simulink model "qdr_ct_test"  (R2012b)
settings: Solver=ode45  StartTime=0.0  StopTime=50000  RelTol=1e-3
libraries: xbsIndex_r4 x1070, casper_library_misc x5, xps_library x4, casper_library_delays x4
(part 2 of 10)

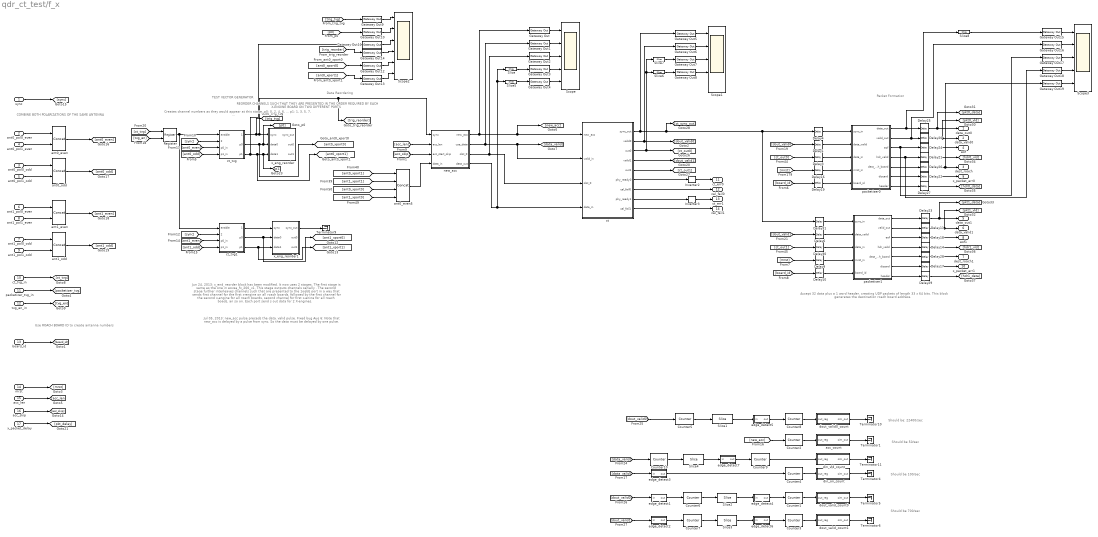
== system qdr_ct_test/f_x ==
  note: Accept 32 data plus a 1 word header,
      | creating UDP packets of length 33 x 64 bits.
      | This block generates the destination roach board address.
  note: Packet Formation
  note: Data Reordering
  note: COMBINE BOTH POLARIZATIONS
      | OF THE SAME ANTENNA
  note: REORDER CHANNELS SUCH THAT
      | THEY ARE PRESENTED IN THE ORDER
      | REQUIRED BY EACH X-ENGINE BOARD
      | ON TWO DIFFERENT PORTS
  note: TEST VECTOR
      | GENERATOR
  note: Creates channel numbers as they
      | would appear at this stage.
      | p0: 0, 2, 4, 6, ...
      | p1: 1, 3, 5, 7, ...
  note: Jun 24, 2013: x_end_reorder block has been modified.
      | It now uses 2 stages. The first stage is same as the one in eovsa_fx_200_v1.
      | This stage outputs channels serially .
      | The second stage further interleaves channels such that are presented to the 1ogbE port in a way that sends first channel for the first x-engine on all roach boards, followed by
      | the first channel for the second x-engine for all roach boards, second channel for first x-enine for all roach boads, an so on. Each port send s out data for 2 X-engines.
  note: Use ROACH BOARD ID to create antenna numbers
  note: Jul 05, 2013: new_acc  pulse preceds the data_valid pulse. Fixed bug
      | Aug 6: Note that new_acc is delayed by a pulse from sync. So the data must be delayed by one pulse.
  note: Should be 50/sec
  note: Should be:
      | 22400/sec
  note: Should be 100/sec
  note: Should be 700/sec
  sync : Inport
  ant0_pol0_even : Inport  Port=2
  ant0_pol0_odd : Inport  Port=3
  ant0_pol1_even : Inport  Port=4
  ant0_pol1_odd : Inport  Port=5
  ant1_pol0_even : Inport  Port=6
  ant1_pol0_odd : Inport  Port=7
  ant1_pol1_even : Inport  Port=8
  ant1_pol1_odd : Inport  Port=9
  ct_tvg_in : Inport  Port=10
  packetizer_tvg_in : Inport  Port=11
  tvg_en_in : Inport  Port=12
  board_id : Inport  Port=13
  mrst : Inport  Port=14
  acc_len : Inport  Port=15
  acc_skip : Inport  Port=16
  x_packet_delay : Inport  Port=17
  Counter{1..4,8..9} (6 alike) : xbsIndex_r4/Counter  cnt_type=Free Running  cnt_to=Inf  operation=Up  start_count=0  cnt_by_val=1  arith_type=Unsigned  n_bits=32  bin_pt=0  load_pin=off  rst=off  en=on  explicit_period=off  period=1  dbl_ovrd=off  use_behavioral_HDL=off  implementation=Fabric  block_type=counter
      settings: block_version=11.4
  Counter10 : xbsIndex_r4/Counter  cnt_type=Free Running  cnt_to=Inf  operation=Up  start_count=0  cnt_by_val=1  arith_type=Unsigned  n_bits=18  bin_pt=0  load_pin=off  rst=off  en=on  explicit_period=off  period=1  dbl_ovrd=off  use_behavioral_HDL=off  implementation=Fabric  block_type=counter
      settings: block_version=11.4
  Counter5 : xbsIndex_r4/Counter  cnt_type=Free Running  cnt_to=Inf  operation=Up  start_count=0  cnt_by_val=1  arith_type=Unsigned  n_bits=12  bin_pt=0  load_pin=off  rst=off  en=on  explicit_period=off  period=1  dbl_ovrd=off  use_behavioral_HDL=off  implementation=Fabric  block_type=counter
      settings: block_version=11.4
  Counter6 : xbsIndex_r4/Counter  cnt_type=Free Running  cnt_to=Inf  operation=Up  start_count=0  cnt_by_val=1  arith_type=Unsigned  n_bits=13  bin_pt=0  load_pin=off  rst=off  en=on  explicit_period=off  period=1  dbl_ovrd=off  use_behavioral_HDL=off  implementation=Fabric  block_type=counter
      settings: block_version=11.4
  Counter7 : xbsIndex_r4/Counter  cnt_type=Free Running  cnt_to=Inf  operation=Up  start_count=0  cnt_by_val=1  arith_type=Unsigned  n_bits=13  bin_pt=0  load_pin=off  rst=off  en=on  explicit_period=off  period=1  dbl_ovrd=off  use_behavioral_HDL=off  implementation=Fabric  block_type=counter
      settings: block_version=11.4
  Delay{1,3..4,6,9..11,14,16..31} (24 alike) : xbsIndex_r4/Delay  rst=off  infoeditControl=Selection of Reset will increase slice count due to use of real FFs and instead of SRLs  en=off  latency=1  dbl_ovrd=off  reg_retiming=on  block_type=delay
      settings: xl_area=[0, 0, 0, 0, 0, 0, 0]
  Gateway Out{,1..19} (20 alike) : xbsIndex_r4/Gateway Out  inherit_from_input=off  hdl_port=on  timing_constraint=None  locs_specified=off  LOCs={}  UseAsDAC=off  DACChannel='1'  block_type=gatewayout
  Inverter2 : xbsIndex_r4/Inverter  en=off  latency=0  dbl_ovrd=off  block_type=inv
      settings: block_version=11.4
  Inverter3 : xbsIndex_r4/Inverter  en=off  latency=0  dbl_ovrd=off  block_type=inv
      settings: block_version=11.4
  Register : xbsIndex_r4/Register  init=0  rst=off  en=on  dbl_ovrd=off  block_type=register
      settings: block_version=11.4
  Scope : Scope  NumInputPorts=5
      settings: YMin=-5~-5~-5~-5~-5  YMax=5~5~5~5~5  SaveName=ScopeData2
  Scope1 : Scope  NumInputPorts=5
      settings: YMin=-5~-5~-5~-5~-5  YMax=5~5~5~5~5  SaveName=ScopeData5
  Scope2 : Scope  NumInputPorts=6
      settings: YMin=-5~-5~-5~-5~-5~-5  YMax=5~5~5~5~5~5
  Scope3 : Scope  NumInputPorts=5
      settings: YMin=-5~-5~-5~-5~-5  YMax=5~5~5~5~5  SaveName=ScopeData6
  Slice : xbsIndex_r4/Slice  nbits=16  boolean_output=off  mode=Lower Bit Location + Width  bit1=0  base1=MSB of Input  bit0=0  base0=LSB of Input  dbl_ovrd=off  block_type=slice
  Slice{1..4} (4 alike) : xbsIndex_r4/Slice  nbits=1  boolean_output=on  mode=Upper Bit Location + Width  bit1=0  base1=MSB of Input  bit0=0  base0=LSB of Input  dbl_ovrd=off  block_type=slice
  Slice5 : xbsIndex_r4/Slice  nbits=16  boolean_output=off  mode=Lower Bit Location + Width  bit1=0  base1=MSB of Input  bit0=16  base0=LSB of Input  dbl_ovrd=off  block_type=slice
  Slice6 : xbsIndex_r4/Slice  nbits=16  boolean_output=off  mode=Lower Bit Location + Width  bit1=0  base1=MSB of Input  bit0=0  base0=LSB of Input  dbl_ovrd=off  block_type=slice
  Slice7 : xbsIndex_r4/Slice  nbits=16  boolean_output=off  mode=Lower Bit Location + Width  bit1=0  base1=MSB of Input  bit0=16  base0=LSB of Input  dbl_ovrd=off  block_type=slice
  Slice8 : xbsIndex_r4/Slice  nbits=16  boolean_output=off  mode=Lower Bit Location + Width  bit1=0  base1=MSB of Input  bit0=0  base0=LSB of Input  dbl_ovrd=off  block_type=slice
  Terminator{1,4..6,9..11} (7 alike) : Terminator
  acc_count : Subsystem  Tag=xps:sw_reg  AncestorBlock=xps_library/software_register  mask(swreg){mode=one value, io_dir=To Processor, io_delay=0, sample_period=1, names=reg, bitwidths=32, arith_types=0, bin_pts=0, sim_port=on, show_format=off}
      mask prompts: io_dir "I/O direction"; io_delay "I/O delay"; sample_period "Sample period"; names "Name:"; bitwidths "Bitwidth:"; arith_types "Type (ufix=0, fix=1, bool=2):"; bin_pts "Binary pt:"; sim_port "Provide sim input/output?"; show_format "Print format string?"
      mask init:
      | swreg_init(gcb)
      settings: AttributesFormatString=1output
      mask TypeOptions mode: one value | fields of equal size | fields of arbitrary size
      mask Callback mode: swreg_cb(gcb);
      mask TypeOptions io_dir: To Processor | From Processor
      mask Callback io_dir:
      | mask_enables = get_param(gcb, 'MaskEnables');
      | mask_names = get_param(gcb, 'MaskNames');
      | if strcmp(get_param(gcb, 'io_dir'), 'To Processor'),
      |     mask_enables{ismember(mask_names, 'sample_period')} = 'off';
      | else
      |     mask_enables{ismember(mask_names, 'sample_period')} = 'on';
      | end
      | set_param(gcb, 'MaskEnables', mask_enables);
      mask Callback bitwidths:
      | swreg_maskcheck(gcb);
      | % blk = gcb;
      | % mode = get_param(blk, 'mode');
      | % current_widths = eval(get_param(blk, 'bitwidths'));
      | % if (strcmp(mode, 'one value') || strcmp(mode, 'fields of equal size')) && (length(current_widths) > 1),
      | %     error('Only one width may be specified for this mode.');
      | % elseif strcmp(mode, 'fields of arbitrary size')
      | %     current_names = textscan(strtrim(strrep(strrep(get_param(blk, 'names'), ']', ''), '[', '')), '%s');
      | %     current_names = current_names{1};
      | %     numios = length(current_names);
      | %     if length(current_widths) ~= numios,
      | %         error('%d field names specified, but %d widths?', numios, length(current_widths));
      | %     end
      | % end
      | % total_width = 0;
      | % for ctr = 1 : length(current_widths),
      | %     total_width = total_width + current_widths(ctr);
      | % end
      | % if total_width > 32,
      | %     error('Total width must be 32 or less, set to %d.', total_width);
      | % end
      mask Callback arith_types:
      | [numios, ~, ~, ~, current_types] = swreg_maskcheck(gcb);
      | % blk = gcb;
      | % mode = get_param(blk, 'mode');
      | % current_types = eval(get_param(blk, 'arith_types'));
      | % numios = length(current_types);
      | % if (strcmp(mode, 'one value') || strcmp(mode, 'fields of equal size')) && (length(current_types) > 1),
      | %     error('Only one type may be specified for this mode.');
      | % elseif strcmp(mode, 'fields of arbitrary size')
      | %     current_names = textscan(strtrim(strrep(strrep(get_param(blk, 'names'), ']', ''), '[', '')), '%s');
      | %     current_names = current_names{1};
      | %     numios = length(current_names);
      | %     if length(current_types) ~= numios,
      | %         error('%d field names specified, but %d types?', numios, length(current_types));
      | %     end
      | % end
      | problem = 0;
      | for ctr = 1 : numios,
      |     t = current_types(ctr);
      |     if (t < 0) || (t > 2),
      |         problem = t;
      |         ctr = numios + 1;
      |     end
      | end
      | if problem ~= 0,
      |     error('Type cannot be %i, must be 0, 1 or 2.', problem);
      | end
      mask Callback bin_pts:
      | swreg_maskcheck(gcb);
      | % blk = gcb;
      | % mode = get_param(blk, 'mode');
      | % current_bins = eval(get_param(blk, 'bin_pts'));
      | % if (strcmp(mode, 'one value') || strcmp(mode, 'fields of equal size')) && (length(current_bins) > 1),
      | %     error('Only one binary pt may be specified for this mode.');
      | % elseif strcmp(mode, 'fields of arbitrary size')
      | %     current_names = textscan(strtrim(strrep(strrep(get_param(blk, 'names'), ']', ''), '[', '')), '%s');
      | %     current_names = current_names{1};
      | %     numios = length(current_names);
      | %     if length(current_bins) ~= numios,
      | %         error('%d field names specified, but %d binary pts?', numios, length(current_bins));
      | %     end
      | % end
  ant0_even : xbsIndex_r4/Concat  num_inputs=2  dbl_ovrd=off  block_type=concat
  ant0_even5 : xbsIndex_r4/Concat  num_inputs=4  dbl_ovrd=off  block_type=concat
  ant0_odd : xbsIndex_r4/Concat  num_inputs=2  dbl_ovrd=off  block_type=concat
  ant1_even : xbsIndex_r4/Concat  num_inputs=2  dbl_ovrd=off  block_type=concat
  ant1_odd : xbsIndex_r4/Concat  num_inputs=2  dbl_ovrd=off  block_type=concat
  ct : Subsystem  mask{freq_chan=fft_size, x_acc_len=5, bram_latency=3, ip_bits=16}
      mask prompts: freq_chan "No. of frequency channels (2 ^ ?)"; x_acc_len "X-eng Accumulation length (2^? samples):"; bram_latency "bram latency"; ip_bits "Input channel bitwidth"
  ct_tvg : Subsystem  mask{num_channels_bits=fft_size, channel_bits=8, ant=0}
      mask prompts: num_channels_bits "Number of channels (2^?):"; channel_bits "Bits per channel:"; ant "Antenna # [0, 15]"
  ct_tvg1 : Subsystem  mask{num_channels_bits=fft_size, channel_bits=8, ant=1}
      mask prompts: num_channels_bits "Number of channels (2^?):"; channel_bits "Bits per channel:"; ant "Antenna # [0, 15]"
  din_on_count : Subsystem  Tag=xps:sw_reg  AncestorBlock=xps_library/software_register  mask(swreg){mode=one value, io_dir=To Processor, io_delay=0, sample_period=1, names=reg, bitwidths=32, arith_types=0, bin_pts=0, sim_port=on, show_format=off}
      mask prompts: io_dir "I/O direction"; io_delay "I/O delay"; sample_period "Sample period"; names "Name:"; bitwidths "Bitwidth:"; arith_types "Type (ufix=0, fix=1, bool=2):"; bin_pts "Binary pt:"; sim_port "Provide sim input/output?"; show_format "Print format string?"
      mask init:
      | swreg_init(gcb)
      settings: AttributesFormatString=1output
      mask TypeOptions mode: one value | fields of equal size | fields of arbitrary size
      mask Callback mode: swreg_cb(gcb);
      mask TypeOptions io_dir: To Processor | From Processor
      mask Callback io_dir:
      | mask_enables = get_param(gcb, 'MaskEnables');
      | mask_names = get_param(gcb, 'MaskNames');
      | if strcmp(get_param(gcb, 'io_dir'), 'To Processor'),
      |     mask_enables{ismember(mask_names, 'sample_period')} = 'off';
      | else
      |     mask_enables{ismember(mask_names, 'sample_period')} = 'on';
      | end
      | set_param(gcb, 'MaskEnables', mask_enables);
      mask Callback bitwidths:
      | swreg_maskcheck(gcb);
      | % blk = gcb;
      | % mode = get_param(blk, 'mode');
      | % current_widths = eval(get_param(blk, 'bitwidths'));
      | % if (strcmp(mode, 'one value') || strcmp(mode, 'fields of equal size')) && (length(current_widths) > 1),
      | %     error('Only one width may be specified for this mode.');
      | % elseif strcmp(mode, 'fields of arbitrary size')
      | %     current_names = textscan(strtrim(strrep(strrep(get_param(blk, 'names'), ']', ''), '[', '')), '%s');
      | %     current_names = current_names{1};
      | %     numios = length(current_names);
      | %     if length(current_widths) ~= numios,
      | %         error('%d field names specified, but %d widths?', numios, length(current_widths));
      | %     end
      | % end
      | % total_width = 0;
      | % for ctr = 1 : length(current_widths),
      | %     total_width = total_width + current_widths(ctr);
      | % end
      | % if total_width > 32,
      | %     error('Total width must be 32 or less, set to %d.', total_width);
      | % end
      mask Callback arith_types:
      | [numios, ~, ~, ~, current_types] = swreg_maskcheck(gcb);
      | % blk = gcb;
      | % mode = get_param(blk, 'mode');
      | % current_types = eval(get_param(blk, 'arith_types'));
      | % numios = length(current_types);
      | % if (strcmp(mode, 'one value') || strcmp(mode, 'fields of equal size')) && (length(current_types) > 1),
      | %     error('Only one type may be specified for this mode.');
      | % elseif strcmp(mode, 'fields of arbitrary size')
      | %     current_names = textscan(strtrim(strrep(strrep(get_param(blk, 'names'), ']', ''), '[', '')), '%s');
      | %     current_names = current_names{1};
      | %     numios = length(current_names);
      | %     if length(current_types) ~= numios,
      | %         error('%d field names specified, but %d types?', numios, length(current_types));
      | %     end
      | % end
      | problem = 0;
      | for ctr = 1 : numios,
      |     t = current_types(ctr);
      |     if (t < 0) || (t > 2),
      |         problem = t;
      |         ctr = numios + 1;
      |     end
      | end
      | if problem ~= 0,
      |     error('Type cannot be %i, must be 0, 1 or 2.', problem);
      | end
      mask Callback bin_pts:
      | swreg_maskcheck(gcb);
      | % blk = gcb;
      | % mode = get_param(blk, 'mode');
      | % current_bins = eval(get_param(blk, 'bin_pts'));
      | % if (strcmp(mode, 'one value') || strcmp(mode, 'fields of equal size')) && (length(current_bins) > 1),
      | %     error('Only one binary pt may be specified for this mode.');
      | % elseif strcmp(mode, 'fields of arbitrary size')
      | %     current_names = textscan(strtrim(strrep(strrep(get_param(blk, 'names'), ']', ''), '[', '')), '%s');
      | %     current_names = current_names{1};
      | %     numios = length(current_names);
      | %     if length(current_bins) ~= numios,
      | %         error('%d field names specified, but %d binary pts?', numios, length(current_bins));
      | %     end
      | % end
  din_vld_count : Subsystem  Tag=xps:sw_reg  AncestorBlock=xps_library/software_register  mask(swreg){mode=one value, io_dir=To Processor, io_delay=0, sample_period=1, names=reg, bitwidths=32, arith_types=0, bin_pts=0, sim_port=on, show_format=off}
      mask prompts: io_dir "I/O direction"; io_delay "I/O delay"; sample_period "Sample period"; names "Name:"; bitwidths "Bitwidth:"; arith_types "Type (ufix=0, fix=1, bool=2):"; bin_pts "Binary pt:"; sim_port "Provide sim input/output?"; show_format "Print format string?"
      mask init:
      | swreg_init(gcb)
      settings: AttributesFormatString=1output
      mask TypeOptions mode: one value | fields of equal size | fields of arbitrary size
      mask Callback mode: swreg_cb(gcb);
      mask TypeOptions io_dir: To Processor | From Processor
      mask Callback io_dir:
      | mask_enables = get_param(gcb, 'MaskEnables');
      | mask_names = get_param(gcb, 'MaskNames');
      | if strcmp(get_param(gcb, 'io_dir'), 'To Processor'),
      |     mask_enables{ismember(mask_names, 'sample_period')} = 'off';
      | else
      |     mask_enables{ismember(mask_names, 'sample_period')} = 'on';
      | end
      | set_param(gcb, 'MaskEnables', mask_enables);
      mask Callback bitwidths:
      | swreg_maskcheck(gcb);
      | % blk = gcb;
      | % mode = get_param(blk, 'mode');
      | % current_widths = eval(get_param(blk, 'bitwidths'));
      | % if (strcmp(mode, 'one value') || strcmp(mode, 'fields of equal size')) && (length(current_widths) > 1),
      | %     error('Only one width may be specified for this mode.');
      | % elseif strcmp(mode, 'fields of arbitrary size')
      | %     current_names = textscan(strtrim(strrep(strrep(get_param(blk, 'names'), ']', ''), '[', '')), '%s');
      | %     current_names = current_names{1};
      | %     numios = length(current_names);
      | %     if length(current_widths) ~= numios,
      | %         error('%d field names specified, but %d widths?', numios, length(current_widths));
      | %     end
      | % end
      | % total_width = 0;
      | % for ctr = 1 : length(current_widths),
      | %     total_width = total_width + current_widths(ctr);
      | % end
      | % if total_width > 32,
      | %     error('Total width must be 32 or less, set to %d.', total_width);
      | % end
      mask Callback arith_types:
      | [numios, ~, ~, ~, current_types] = swreg_maskcheck(gcb);
      | % blk = gcb;
      | % mode = get_param(blk, 'mode');
      | % current_types = eval(get_param(blk, 'arith_types'));
      | % numios = length(current_types);
      | % if (strcmp(mode, 'one value') || strcmp(mode, 'fields of equal size')) && (length(current_types) > 1),
      | %     error('Only one type may be specified for this mode.');
      | % elseif strcmp(mode, 'fields of arbitrary size')
      | %     current_names = textscan(strtrim(strrep(strrep(get_param(blk, 'names'), ']', ''), '[', '')), '%s');
      | %     current_names = current_names{1};
      | %     numios = length(current_names);
      | %     if length(current_types) ~= numios,
      | %         error('%d field names specified, but %d types?', numios, length(current_types));
      | %     end
      | % end
      | problem = 0;
      | for ctr = 1 : numios,
      |     t = current_types(ctr);
      |     if (t < 0) || (t > 2),
      |         problem = t;
      |         ctr = numios + 1;
      |     end
      | end
      | if problem ~= 0,
      |     error('Type cannot be %i, must be 0, 1 or 2.', problem);
      | end
      mask Callback bin_pts:
      | swreg_maskcheck(gcb);
      | % blk = gcb;
      | % mode = get_param(blk, 'mode');
      | % current_bins = eval(get_param(blk, 'bin_pts'));
      | % if (strcmp(mode, 'one value') || strcmp(mode, 'fields of equal size')) && (length(current_bins) > 1),
      | %     error('Only one binary pt may be specified for this mode.');
      | % elseif strcmp(mode, 'fields of arbitrary size')
      | %     current_names = textscan(strtrim(strrep(strrep(get_param(blk, 'names'), ']', ''), '[', '')), '%s');
      | %     current_names = current_names{1};
      | %     numios = length(current_names);
      | %     if length(current_bins) ~= numios,
      | %         error('%d field names specified, but %d binary pts?', numios, length(current_bins));
      | %     end
      | % end
  dout_valid0_count : Subsystem  Tag=xps:sw_reg  AncestorBlock=xps_library/software_register  mask(swreg){mode=one value, io_dir=To Processor, io_delay=0, sample_period=1, names=reg, bitwidths=32, arith_types=0, bin_pts=0, sim_port=on, show_format=off}
      mask prompts: io_dir "I/O direction"; io_delay "I/O delay"; sample_period "Sample period"; names "Name:"; bitwidths "Bitwidth:"; arith_types "Type (ufix=0, fix=1, bool=2):"; bin_pts "Binary pt:"; sim_port "Provide sim input/output?"; show_format "Print format string?"
      mask init:
      | swreg_init(gcb)
      settings: AttributesFormatString=1output
      mask TypeOptions mode: one value | fields of equal size | fields of arbitrary size
      mask Callback mode: swreg_cb(gcb);
      mask TypeOptions io_dir: To Processor | From Processor
      mask Callback io_dir:
      | mask_enables = get_param(gcb, 'MaskEnables');
      | mask_names = get_param(gcb, 'MaskNames');
      | if strcmp(get_param(gcb, 'io_dir'), 'To Processor'),
      |     mask_enables{ismember(mask_names, 'sample_period')} = 'off';
      | else
      |     mask_enables{ismember(mask_names, 'sample_period')} = 'on';
      | end
      | set_param(gcb, 'MaskEnables', mask_enables);
      mask Callback bitwidths:
      | swreg_maskcheck(gcb);
      | % blk = gcb;
      | % mode = get_param(blk, 'mode');
      | % current_widths = eval(get_param(blk, 'bitwidths'));
      | % if (strcmp(mode, 'one value') || strcmp(mode, 'fields of equal size')) && (length(current_widths) > 1),
      | %     error('Only one width may be specified for this mode.');
      | % elseif strcmp(mode, 'fields of arbitrary size')
      | %     current_names = textscan(strtrim(strrep(strrep(get_param(blk, 'names'), ']', ''), '[', '')), '%s');
      | %     current_names = current_names{1};
      | %     numios = length(current_names);
      | %     if length(current_widths) ~= numios,
      | %         error('%d field names specified, but %d widths?', numios, length(current_widths));
      | %     end
      | % end
      | % total_width = 0;
      | % for ctr = 1 : length(current_widths),
      | %     total_width = total_width + current_widths(ctr);
      | % end
      | % if total_width > 32,
      | %     error('Total width must be 32 or less, set to %d.', total_width);
      | % end
      mask Callback arith_types:
      | [numios, ~, ~, ~, current_types] = swreg_maskcheck(gcb);
      | % blk = gcb;
      | % mode = get_param(blk, 'mode');
      | % current_types = eval(get_param(blk, 'arith_types'));
      | % numios = length(current_types);
      | % if (strcmp(mode, 'one value') || strcmp(mode, 'fields of equal size')) && (length(current_types) > 1),
      | %     error('Only one type may be specified for this mode.');
      | % elseif strcmp(mode, 'fields of arbitrary size')
      | %     current_names = textscan(strtrim(strrep(strrep(get_param(blk, 'names'), ']', ''), '[', '')), '%s');
      | %     current_names = current_names{1};
      | %     numios = length(current_names);
      | %     if length(current_types) ~= numios,
      | %         error('%d field names specified, but %d types?', numios, length(current_types));
      | %     end
      | % end
      | problem = 0;
      | for ctr = 1 : numios,
      |     t = current_types(ctr);
      |     if (t < 0) || (t > 2),
      |         problem = t;
      |         ctr = numios + 1;
      |     end
      | end
      | if problem ~= 0,
      |     error('Type cannot be %i, must be 0, 1 or 2.', problem);
      | end
      mask Callback bin_pts:
      | swreg_maskcheck(gcb);
      | % blk = gcb;
      | % mode = get_param(blk, 'mode');
      | % current_bins = eval(get_param(blk, 'bin_pts'));
      | % if (strcmp(mode, 'one value') || strcmp(mode, 'fields of equal size')) && (length(current_bins) > 1),
      | %     error('Only one binary pt may be specified for this mode.');
      | % elseif strcmp(mode, 'fields of arbitrary size')
      | %     current_names = textscan(strtrim(strrep(strrep(get_param(blk, 'names'), ']', ''), '[', '')), '%s');
      | %     current_names = current_names{1};
      | %     numios = length(current_names);
      | %     if length(current_bins) ~= numios,
      | %         error('%d field names specified, but %d binary pts?', numios, length(current_bins));
      | %     end
      | % end
  dout_valid_count0 : Subsystem  Tag=xps:sw_reg  AncestorBlock=xps_library/software_register  mask(swreg){mode=one value, io_dir=To Processor, io_delay=0, sample_period=1, names=reg, bitwidths=32, arith_types=0, bin_pts=0, sim_port=on, show_format=off}
      mask prompts: io_dir "I/O direction"; io_delay "I/O delay"; sample_period "Sample period"; names "Name:"; bitwidths "Bitwidth:"; arith_types "Type (ufix=0, fix=1, bool=2):"; bin_pts "Binary pt:"; sim_port "Provide sim input/output?"; show_format "Print format string?"
      mask init:
      | swreg_init(gcb)
      settings: AttributesFormatString=1output
      mask TypeOptions mode: one value | fields of equal size | fields of arbitrary size
      mask Callback mode: swreg_cb(gcb);
      mask TypeOptions io_dir: To Processor | From Processor
      mask Callback io_dir:
      | mask_enables = get_param(gcb, 'MaskEnables');
      | mask_names = get_param(gcb, 'MaskNames');
      | if strcmp(get_param(gcb, 'io_dir'), 'To Processor'),
      |     mask_enables{ismember(mask_names, 'sample_period')} = 'off';
      | else
      |     mask_enables{ismember(mask_names, 'sample_period')} = 'on';
      | end
      | set_param(gcb, 'MaskEnables', mask_enables);
      mask Callback bitwidths:
      | swreg_maskcheck(gcb);
      | % blk = gcb;
      | % mode = get_param(blk, 'mode');
      | % current_widths = eval(get_param(blk, 'bitwidths'));
      | % if (strcmp(mode, 'one value') || strcmp(mode, 'fields of equal size')) && (length(current_widths) > 1),
      | %     error('Only one width may be specified for this mode.');
      | % elseif strcmp(mode, 'fields of arbitrary size')
      | %     current_names = textscan(strtrim(strrep(strrep(get_param(blk, 'names'), ']', ''), '[', '')), '%s');
      | %     current_names = current_names{1};
      | %     numios = length(current_names);
      | %     if length(current_widths) ~= numios,
      | %         error('%d field names specified, but %d widths?', numios, length(current_widths));
      | %     end
      | % end
      | % total_width = 0;
      | % for ctr = 1 : length(current_widths),
      | %     total_width = total_width + current_widths(ctr);
      | % end
      | % if total_width > 32,
      | %     error('Total width must be 32 or less, set to %d.', total_width);
      | % end
      mask Callback arith_types:
      | [numios, ~, ~, ~, current_types] = swreg_maskcheck(gcb);
      | % blk = gcb;
      | % mode = get_param(blk, 'mode');
      | % current_types = eval(get_param(blk, 'arith_types'));
      | % numios = length(current_types);
      | % if (strcmp(mode, 'one value') || strcmp(mode, 'fields of equal size')) && (length(current_types) > 1),
      | %     error('Only one type may be specified for this mode.');
      | % elseif strcmp(mode, 'fields of arbitrary size')
      | %     current_names = textscan(strtrim(strrep(strrep(get_param(blk, 'names'), ']', ''), '[', '')), '%s');
      | %     current_names = current_names{1};
      | %     numios = length(current_names);
      | %     if length(current_types) ~= numios,
      | %         error('%d field names specified, but %d types?', numios, length(current_types));
      | %     end
      | % end
      | problem = 0;
      | for ctr = 1 : numios,
      |     t = current_types(ctr);
      |     if (t < 0) || (t > 2),
      |         problem = t;
      |         ctr = numios + 1;
      |     end
      | end
      | if problem ~= 0,
      |     error('Type cannot be %i, must be 0, 1 or 2.', problem);
      | end
      mask Callback bin_pts:
      | swreg_maskcheck(gcb);
      | % blk = gcb;
      | % mode = get_param(blk, 'mode');
      | % current_bins = eval(get_param(blk, 'bin_pts'));
      | % if (strcmp(mode, 'one value') || strcmp(mode, 'fields of equal size')) && (length(current_bins) > 1),
      | %     error('Only one binary pt may be specified for this mode.');
      | % elseif strcmp(mode, 'fields of arbitrary size')
      | %     current_names = textscan(strtrim(strrep(strrep(get_param(blk, 'names'), ']', ''), '[', '')), '%s');
      | %     current_names = current_names{1};
      | %     numios = length(current_names);
      | %     if length(current_bins) ~= numios,
      | %         error('%d field names specified, but %d binary pts?', numios, length(current_bins));
      | %     end
      | % end
  dout_valid_count1 : Subsystem  Tag=xps:sw_reg  AncestorBlock=xps_library/software_register  mask(swreg){mode=one value, io_dir=To Processor, io_delay=0, sample_period=1, names=reg, bitwidths=32, arith_types=0, bin_pts=0, sim_port=on, show_format=off}
      mask prompts: io_dir "I/O direction"; io_delay "I/O delay"; sample_period "Sample period"; names "Name:"; bitwidths "Bitwidth:"; arith_types "Type (ufix=0, fix=1, bool=2):"; bin_pts "Binary pt:"; sim_port "Provide sim input/output?"; show_format "Print format string?"
      mask init:
      | swreg_init(gcb)
      settings: AttributesFormatString=1output
      mask TypeOptions mode: one value | fields of equal size | fields of arbitrary size
      mask Callback mode: swreg_cb(gcb);
      mask TypeOptions io_dir: To Processor | From Processor
      mask Callback io_dir:
      | mask_enables = get_param(gcb, 'MaskEnables');
      | mask_names = get_param(gcb, 'MaskNames');
      | if strcmp(get_param(gcb, 'io_dir'), 'To Processor'),
      |     mask_enables{ismember(mask_names, 'sample_period')} = 'off';
      | else
      |     mask_enables{ismember(mask_names, 'sample_period')} = 'on';
      | end
      | set_param(gcb, 'MaskEnables', mask_enables);
      mask Callback bitwidths:
      | swreg_maskcheck(gcb);
      | % blk = gcb;
      | % mode = get_param(blk, 'mode');
      | % current_widths = eval(get_param(blk, 'bitwidths'));
      | % if (strcmp(mode, 'one value') || strcmp(mode, 'fields of equal size')) && (length(current_widths) > 1),
      | %     error('Only one width may be specified for this mode.');
      | % elseif strcmp(mode, 'fields of arbitrary size')
      | %     current_names = textscan(strtrim(strrep(strrep(get_param(blk, 'names'), ']', ''), '[', '')), '%s');
      | %     current_names = current_names{1};
      | %     numios = length(current_names);
      | %     if length(current_widths) ~= numios,
      | %         error('%d field names specified, but %d widths?', numios, length(current_widths));
      | %     end
      | % end
      | % total_width = 0;
      | % for ctr = 1 : length(current_widths),
      | %     total_width = total_width + current_widths(ctr);
      | % end
      | % if total_width > 32,
      | %     error('Total width must be 32 or less, set to %d.', total_width);
      | % end
      mask Callback arith_types:
      | [numios, ~, ~, ~, current_types] = swreg_maskcheck(gcb);
      | % blk = gcb;
      | % mode = get_param(blk, 'mode');
      | % current_types = eval(get_param(blk, 'arith_types'));
      | % numios = length(current_types);
      | % if (strcmp(mode, 'one value') || strcmp(mode, 'fields of equal size')) && (length(current_types) > 1),
      | %     error('Only one type may be specified for this mode.');
      | % elseif strcmp(mode, 'fields of arbitrary size')
      | %     current_names = textscan(strtrim(strrep(strrep(get_param(blk, 'names'), ']', ''), '[', '')), '%s');
      | %     current_names = current_names{1};
      | %     numios = length(current_names);
      | %     if length(current_types) ~= numios,
      | %         error('%d field names specified, but %d types?', numios, length(current_types));
      | %     end
      | % end
      | problem = 0;
      | for ctr = 1 : numios,
      |     t = current_types(ctr);
      |     if (t < 0) || (t > 2),
      |         problem = t;
      |         ctr = numios + 1;
      |     end
      | end
      | if problem ~= 0,
      |     error('Type cannot be %i, must be 0, 1 or 2.', problem);
      | end
      mask Callback bin_pts:
      | swreg_maskcheck(gcb);
      | % blk = gcb;
      | % mode = get_param(blk, 'mode');
      | % current_bins = eval(get_param(blk, 'bin_pts'));
      | % if (strcmp(mode, 'one value') || strcmp(mode, 'fields of equal size')) && (length(current_bins) > 1),
      | %     error('Only one binary pt may be specified for this mode.');
      | % elseif strcmp(mode, 'fields of arbitrary size')
      | %     current_names = textscan(strtrim(strrep(strrep(get_param(blk, 'names'), ']', ''), '[', '')), '%s');
      | %     current_names = current_names{1};
      | %     numios = length(current_names);
      | %     if length(current_bins) ~= numios,
      | %         error('%d field names specified, but %d binary pts?', numios, length(current_bins));
      | %     end
      | % end
  edge_detect1 : Subsystem  AncestorBlock=casper_library_misc/edge_detect  mask(edge_detect){edge=Both, polarity=Active High, x_in=[0 0.08 0.08 0.16 0.16 0.24 0.24 0.32 0.32 0.4], y_in=[-1 -1  1  1  1  1 -1 -1 -1 -1], x_out=[0.6 0.68 0.68 0.76 0.76 0.84 0.84 0.92 0.92 1], y_out=[-1 -1  1  1 -1 -1  1  1 -1 -1]}
      mask prompts: edge "Edge Type"; polarity "Output Polarity"; x_in "Input X Positions"; y_in "Input Y Positions"; x_out "Output X Positions"; y_out "Output Y Positions"
      mask help: Output is active for one-cycle after each edge of the specified type (i.e. rising, falling or both).
      mask init:
      | edge_detect_init(gcb,...
      |     'edge',edge,...
      |     'polarity',polarity,...
      |     'x_in',x_in,...
      |     'x_out',x_out,...
      |     'y_in',y_in,...
      |     'y_out',y_out);
      | 
      | x_in_num=str2num(getfield(getfield(get_param(gcb,'UserData'),'parameters'),'x_in'));
      | x_out_num=str2num(getfield(getfield(get_param(gcb,'UserData'),'parameters'),'x_out'));
      | y_in_num=str2num(getfield(getfield(get_param(gcb,'UserData'),'parameters'),'y_in'));
      | y_out_num=str2num(getfield(getfield(get_param(gcb,'UserData'),'parameters'),'y_out'));
      settings: AttributesFormatString=|
      | both edges
      | active high
      mask Help: Output is active for one-cycle after each edge of the specified type (i.e. rising, falling, or both).  Latency is zero.
      mask TypeOptions edge: Rising | Falling | Both
      mask TypeOptions polarity: Active High | Active Low
      mask Display:
      | plot(x_in_num,0.5+y_in_num*0.2);
      | plot(x_out_num,0.5+y_out_num*0.2);
  edge_detect2 : Subsystem  AncestorBlock=casper_library_misc/edge_detect  mask(edge_detect){edge=Both, polarity=Active High, x_in=[0 0.08 0.08 0.16 0.16 0.24 0.24 0.32 0.32 0.4], y_in=[-1 -1  1  1  1  1 -1 -1 -1 -1], x_out=[0.6 0.68 0.68 0.76 0.76 0.84 0.84 0.92 0.92 1], y_out=[-1 -1  1  1 -1 -1  1  1 -1 -1]}
      mask prompts: edge "Edge Type"; polarity "Output Polarity"; x_in "Input X Positions"; y_in "Input Y Positions"; x_out "Output X Positions"; y_out "Output Y Positions"
      mask help: Output is active for one-cycle after each edge of the specified type (i.e. rising, falling or both).
      mask init: same as qdr_ct_test/f_x/edge_detect1
      settings: AttributesFormatString=|
      | both edges
      | active high
      mask Help: Output is active for one-cycle after each edge of the specified type (i.e. rising, falling, or both).  Latency is zero.
      mask TypeOptions edge: Rising | Falling | Both
      mask TypeOptions polarity: Active High | Active Low
      mask Display:
      | plot(x_in_num,0.5+y_in_num*0.2);
      | plot(x_out_num,0.5+y_out_num*0.2);
  edge_detect3 : Subsystem  AncestorBlock=casper_library_misc/edge_detect  mask(edge_detect){edge=Both, polarity=Active High, x_in=[0 0.08 0.08 0.16 0.16 0.24 0.24 0.32 0.32 0.4], y_in=[-1 -1  1  1  1  1 -1 -1 -1 -1], x_out=[0.6 0.68 0.68 0.76 0.76 0.84 0.84 0.92 0.92 1], y_out=[-1 -1  1  1 -1 -1  1  1 -1 -1]}
      mask prompts: edge "Edge Type"; polarity "Output Polarity"; x_in "Input X Positions"; y_in "Input Y Positions"; x_out "Output X Positions"; y_out "Output Y Positions"
      mask help: Output is active for one-cycle after each edge of the specified type (i.e. rising, falling or both).
      mask init: same as qdr_ct_test/f_x/edge_detect1
      settings: AttributesFormatString=|
      | both edges
      | active high
      mask Help: Output is active for one-cycle after each edge of the specified type (i.e. rising, falling, or both).  Latency is zero.
      mask TypeOptions edge: Rising | Falling | Both
      mask TypeOptions polarity: Active High | Active Low
      mask Display:
      | plot(x_in_num,0.5+y_in_num*0.2);
      | plot(x_out_num,0.5+y_out_num*0.2);
  edge_detect4 : Subsystem  AncestorBlock=casper_library_misc/edge_detect  mask(edge_detect){edge=Falling, polarity=Active High, x_in=[0 0.08 0.08 0.16 0.16 0.24 0.24 0.32 0.32 0.4], y_in=[1  1 -1 -1 -1 -1 -1 -1 -1 -1], x_out=[0.6 0.68 0.68 0.76 0.76 0.84 0.84 0.92 0.92 1], y_out=[-1 -1  1  1 -1 -1 -1 -1 -1 -1]}
      mask prompts: edge "Edge Type"; polarity "Output Polarity"; x_in "Input X Positions"; y_in "Input Y Positions"; x_out "Output X Positions"; y_out "Output Y Positions"
      mask help: Output is active for one-cycle after each edge of the specified type (i.e. rising, falling or both).
      mask init: same as qdr_ct_test/f_x/edge_detect1
      settings: AttributesFormatString=|
      | falling edges
      | active high
      mask Help: Output is active for one-cycle after each edge of the specified type (i.e. rising, falling, or both).  Latency is zero.
      mask TypeOptions edge: Rising | Falling | Both
      mask TypeOptions polarity: Active High | Active Low
      mask Display:
      | plot(x_in_num,0.5+y_in_num*0.2);
      | plot(x_out_num,0.5+y_out_num*0.2);
  edge_detect5 : Subsystem  AncestorBlock=casper_library_misc/edge_detect  mask(edge_detect){edge=Falling, polarity=Active High, x_in=[0 0.08 0.08 0.16 0.16 0.24 0.24 0.32 0.32 0.4], y_in=[1  1 -1 -1 -1 -1 -1 -1 -1 -1], x_out=[0.6 0.68 0.68 0.76 0.76 0.84 0.84 0.92 0.92 1], y_out=[-1 -1  1  1 -1 -1 -1 -1 -1 -1]}
      mask prompts: edge "Edge Type"; polarity "Output Polarity"; x_in "Input X Positions"; y_in "Input Y Positions"; x_out "Output X Positions"; y_out "Output Y Positions"
      mask help: Output is active for one-cycle after each edge of the specified type (i.e. rising, falling or both).
      mask init: same as qdr_ct_test/f_x/edge_detect1
      settings: AttributesFormatString=|
      | falling edges
      | active high
      mask Help: Output is active for one-cycle after each edge of the specified type (i.e. rising, falling, or both).  Latency is zero.
      mask TypeOptions edge: Rising | Falling | Both
      mask TypeOptions polarity: Active High | Active Low
      mask Display:
      | plot(x_in_num,0.5+y_in_num*0.2);
      | plot(x_out_num,0.5+y_out_num*0.2);
  edge_detect6 : Subsystem  AncestorBlock=casper_library_misc/edge_detect  mask(edge_detect){edge=Falling, polarity=Active High, x_in=[0 0.08 0.08 0.16 0.16 0.24 0.24 0.32 0.32 0.4], y_in=[1  1 -1 -1 -1 -1 -1 -1 -1 -1], x_out=[0.6 0.68 0.68 0.76 0.76 0.84 0.84 0.92 0.92 1], y_out=[-1 -1  1  1 -1 -1 -1 -1 -1 -1]}
      mask prompts: edge "Edge Type"; polarity "Output Polarity"; x_in "Input X Positions"; y_in "Input Y Positions"; x_out "Output X Positions"; y_out "Output Y Positions"
      mask help: Output is active for one-cycle after each edge of the specified type (i.e. rising, falling or both).
      mask init: same as qdr_ct_test/f_x/edge_detect1
      settings: AttributesFormatString=|
      | falling edges
      | active high
      mask Help: Output is active for one-cycle after each edge of the specified type (i.e. rising, falling, or both).  Latency is zero.
      mask TypeOptions edge: Rising | Falling | Both
      mask TypeOptions polarity: Active High | Active Low
      mask Display:
      | plot(x_in_num,0.5+y_in_num*0.2);
      | plot(x_out_num,0.5+y_out_num*0.2);
  edge_detect7 : Subsystem  AncestorBlock=casper_library_misc/edge_detect  mask(edge_detect){edge=Falling, polarity=Active High, x_in=[0 0.08 0.08 0.16 0.16 0.24 0.24 0.32 0.32 0.4], y_in=[1  1 -1 -1 -1 -1 -1 -1 -1 -1], x_out=[0.6 0.68 0.68 0.76 0.76 0.84 0.84 0.92 0.92 1], y_out=[-1 -1  1  1 -1 -1 -1 -1 -1 -1]}
      mask prompts: edge "Edge Type"; polarity "Output Polarity"; x_in "Input X Positions"; y_in "Input Y Positions"; x_out "Output X Positions"; y_out "Output Y Positions"
      mask help: Output is active for one-cycle after each edge of the specified type (i.e. rising, falling or both).
      mask init: same as qdr_ct_test/f_x/edge_detect1
      settings: AttributesFormatString=|
      | falling edges
      | active high
      mask Help: Output is active for one-cycle after each edge of the specified type (i.e. rising, falling, or both).  Latency is zero.
      mask TypeOptions edge: Rising | Falling | Both
      mask TypeOptions polarity: Active High | Active Low
      mask Display:
      | plot(x_in_num,0.5+y_in_num*0.2);
      | plot(x_out_num,0.5+y_out_num*0.2);
  new_acc : Subsystem
  packetiser0 : Subsystem  mask{payload_bits=5-2, n_x_board=2, freq_chan=fft_size, n_boards=3, gbe_port=0}
      mask prompts: payload_bits "Payload length in 64bit words (2^?)"; n_x_board "Number of x-engines per ROACH board (2^?)"; freq_chan "Number of frequencies (2^?)"; n_boards "Number of  ROACH boards (2 ^ ?)"; gbe_port "Port # (0 or 1)"
      mask help: Package 32 bit data into 64 bits and identify data as coming from antenna 0 or 1
      mask init:
      | n_x = n_x_board - 1;
  packetiser1 : Subsystem  mask{payload_bits=5, n_x_board=2, freq_chan=fft_size, n_boards=3, gbe_port=1}
      mask prompts: payload_bits "Payload length in 64bit words (2^?)"; n_x_board "Number of x-engines per ROACH board (2^?)"; freq_chan "Number of frequencies (2^?)"; n_boards "Number of  ROACH boards (2 ^ ?)"; gbe_port "Port # (0 or 1)"
      mask help: Package 32 bit data into 64 bits and identify data as coming from antenna 0 or 1
      mask init:
      | n_x = n_x_board - 1;
  x_eng_reorder : Subsystem  mask{freq_chan=fft_size, num_data_bits=16, bram_latency=2, n_boards=3, n_x_board=2}
      mask prompts: freq_chan "Number of Frequency Channels (2 ^ ?)"; num_data_bits "Incomin data width in bits"; bram_latency "BRAM Latency"; n_boards "Number of ROACH boards (2 ^ ?)"; n_x_board "Number of X-engines per ROACH board (2 ^ ?)"
      mask help:
      | Reorders channels for transmission to X-engines in two stages.
      |
      | In the first stage, total of P channels on both inputs (P/2 on each input)
      | are reordered as follows:
      |
      | Input data0 has channels: 0, 2, 4, ..., P-2.
      | Input data1 has channels: 1, 3, 5, ..., P-1.
      | Then,
      | Output out0 has channels: 0, 1, 2, ..., P/2 -1.
      | Output out1 has channels: P/2, P/2 + 1, ..., P-1.
      |
      | Here P = 2 ^ (N - B),
      | where 2 ^ N = no. of total frequency channels
      | and 2 ^ B = total number of ROACH boards
      |
      | In the second stage, the channels on the each output are reordered in a way
      | that when presented to the 10 GbE port, they appear in the following order:
      | First channel to the first X-engine connected to the receiving 10gbE port of all ROACH boards.
      | First channel to the second X-engine connected to the receiving 10GbE port of all ROACH boards.
      | and so on.
      mask init:
      | n_x = n_x_board - 1;
  x_eng_reorder1 : Subsystem  mask{freq_chan=fft_size, num_data_bits=16, bram_latency=2, n_boards=3, n_x_board=2}
      mask prompts: freq_chan "Number of Frequency Channels (2 ^ ?)"; num_data_bits "Incomin data width in bits"; bram_latency "BRAM Latency"; n_boards "Number of ROACH boards (2 ^ ?)"; n_x_board "Number of X-engines per ROACH board (2 ^ ?)"
      mask help:
      | Reorders channels for transmission to X-engines in two stages.
      |
      | In the first stage, total of P channels on both inputs (P/2 on each input)
      | are reordered as follows:
      |
      | Input data0 has channels: 0, 2, 4, ..., P-2.
      | Input data1 has channels: 1, 3, 5, ..., P-1.
      | Then,
      | Output out0 has channels: 0, 1, 2, ..., P/2 -1.
      | Output out1 has channels: P/2, P/2 + 1, ..., P-1.
      |
      | Here P = 2 ^ (N - B),
      | where 2 ^ N = no. of total frequency channels
      | and 2 ^ B = total number of ROACH boards
      |
      | In the second stage, the channels on the each output are reordered in a way
      | that when presented to the 10 GbE port, they appear in the following order:
      | First channel to the first X-engine connected to the receiving 10gbE port of all ROACH boards.
      | First channel to the second X-engine connected to the receiving 10GbE port of all ROACH boards.
      | and so on.
      mask init:
      | n_x = n_x_board - 1;
  data_out0 : Outport
  data_valid0 : Outport  Port=2
  dest_roach : Outport  Port=3
  eof : Outport  Port=4
  data_out1 : Outport  Port=5
  data_valid1 : Outport  Port=6
  dest_roach1 : Outport  Port=7
  eof1 : Outport  Port=8
  x_packet_err0 : Outport  Port=9
  x_packet_err1 : Outport  Port=10
  ct_err0 : Outport  Port=11
  cal_fail0 : Outport  Port=12
  ct_err1 : Outport  Port=13
  cal_fail1 : Outport  Port=14
  wires:
  [ct_tvg] -> Register/1
  [tvg_en] -> Register/2
  Register/1 -> ct_tvg/1(enable), ct_tvg1/1(enable)
  ct_tvg1/1(sync_out) -> x_eng_reorder1/1(sync)
  ct_tvg1/2(p0) -> [ant1_xport0], x_eng_reorder1/2(data0)
  ct_tvg1/3(p1) -> [ant1_xport1], x_eng_reorder1/3(data1)
  ct_tvg_in/1 -> [ct_tvg]
  tvg_en_in/1 -> [tvg_en]
  packetizer_tvg_in/1 -> [packetizer_tvg]
  board_id/1 -> [board_id]
  mrst/1 -> [mrst]
  ant0_pol0_even/1 -> ant0_even/1
  ant0_pol1_even/1 -> ant0_even/2
  ant0_pol0_odd/1 -> ant0_odd/1
  ant0_pol1_odd/1 -> ant0_odd/2
  acc_len/1 -> [acc_len]
  [acc_len] -> new_acc/2(acc_len)
  x_eng_reorder1/1(sync_out) -> Terminator9/1
  ct_tvg/1(sync_out) -> [trig_tvg], [trig_reorder], new_acc/1(sync), x_eng_reorder/1(sync)
  ct_tvg/2(p0) -> [ant0_xport0], [p0], x_eng_reorder/2(data0)
  ct_tvg/3(p1) -> Gateway Out11/1, [ant0_xport1], [p1], x_eng_reorder/3(data1)
  acc_skip/1 -> [acc_skip]
  [acc_skip] -> new_acc/3(acc_start_skip)
  Inverter2/1 -> ct_err0/1
  Inverter3/1 -> ct_err1/1
  ct/1(sync_out) -> Gateway Out5/1, [ct_sync_out], Delay4/1, Delay31/1
  ct/3(out0) -> Slice7/1, Slice6/1, [ct_out0]
  ct/6(phy_ready0) -> Inverter2/1
  ct/7(cal_fail0) -> cal_fail0/1
  ct/8(phy_ready1) -> Inverter3/1
  ant1_pol0_even/1 -> ant1_even/1
  ant1_pol1_even/1 -> ant1_even/2
  ant1_pol0_odd/1 -> ant1_odd/1
  ant1_pol1_odd/1 -> ant1_odd/2
  sync/1 -> [sync]
  ant0_even/1 -> [ant0_even]
  ant0_odd/1 -> [ant0_odd]
  ant1_even/1 -> [ant1_even]
  ant1_odd/1 -> [ant1_odd]
  [sync] -> ct_tvg/2(sync_in)
  [ant0_even] -> ct_tvg/3(p0_in)
  [ant0_odd] -> ct_tvg/4(p1_in)
  [sync] -> ct_tvg1/2(sync_in)
  [ant1_even] -> ct_tvg1/3(p0_in)
  [ant1_odd] -> ct_tvg1/4(p1_in)
  acc_count/1(sim_out) -> Terminator1/1
  [new_acc] -> Counter2/1
  Counter2/1 -> acc_count/1(out_reg)
  din_on_count/1(sim_out) -> Terminator4/1
  Counter4/1 -> din_on_count/1(out_reg)
  [data_valid] -> edge_detect3/1(in)
  edge_detect3/1(out) -> Counter4/1
  dout_valid_count0/1(sim_out) -> Terminator5/1
  Counter1/1 -> dout_valid_count0/1(out_reg)
  edge_detect1/1(out) -> Counter6/1
  dout_valid_count1/1(sim_out) -> Terminator6/1
  Counter3/1 -> dout_valid_count1/1(out_reg)
  ct/2(valid0) -> Gateway Out6/1, [dout_valid0]
  ct/4(valid1) -> [dout_valid1]
  dout_valid0_count/1(sim_out) -> Terminator10/1
  Counter5/1 -> Slice1/1
  edge_detect5/1(out) -> Counter8/1
  Slice1/1 -> edge_detect5/1(in)
  Counter8/1 -> dout_valid0_count/1(out_reg)
  [dout_valid0] -> edge_detect1/1(in)
  [dout_valid1] -> edge_detect2/1(in)
  [dout_valid0] -> Counter5/1
  x_packet_delay/1 -> [pkt_delay]
  Counter6/1 -> Slice2/1
  Slice2/1 -> edge_detect4/1(in)
  edge_detect4/1(out) -> Counter1/1
  Counter7/1 -> Slice3/1
  Slice3/1 -> edge_detect6/1(in)
  edge_detect2/1(out) -> Counter7/1
  edge_detect6/1(out) -> Counter3/1
  ct/5(out1) -> [ct_out1]
  Counter10/1 -> Slice4/1
  Slice4/1 -> edge_detect7/1(in)
  edge_detect7/1(out) -> Counter9/1
  [data_valid] -> Counter10/1
  Counter9/1 -> din_vld_count/1(out_reg)
  din_vld_count/1(sim_out) -> Terminator11/1
  [ant0_xport1] -> ant0_even5/1
  [ant1_xport1] -> ant0_even5/2
  [ant0_xport0] -> ant0_even5/3
  [ant1_xport0] -> ant0_even5/4
  ant0_even5/1 -> new_acc/4(data_in)
  [dout_valid0] -> Delay1/1
  [ct_out0] -> Delay3/1
  [mrst] -> Delay16/1
  [board_id] -> Delay19/1
  Delay4/1 -> packetiser0/1(sync_in)
  Delay1/1 -> packetiser0/2(data_valid)
  Delay3/1 -> packetiser0/3(data_in)
  Delay16/1 -> packetiser0/4(mrst_in)
  Delay19/1 -> packetiser0/5(board_id)
  packetiser0/1(data_out) -> Slice8/1, Delay25/1
  packetiser0/2(valid_out) -> Gateway Out16/1, Delay20/1
  packetiser0/3(eof) -> Gateway Out17/1, Delay24/1
  packetiser0/4(hdr_valid) -> Gateway Out18/1, Delay21/1
  packetiser0/7(header) -> Delay27/1
  packetiser0/5(dest_roach_board) -> Delay26/1
  packetiser0/6(discard) -> Delay22/1
  Delay25/1 -> data_out0/1, [pkt0_data]
  Delay20/1 -> data_valid0/1, [pkt0_vld]
  Delay26/1 -> Gateway Out19/1, dest_roach/1
  Delay24/1 -> eof/1
  Delay22/1 -> x_packet_err0/1
  Delay21/1 -> [hdr0_vld]
  Delay27/1 -> [hdr0_data]
  [dout_valid1] -> Delay6/1
  [ct_out1] -> Delay30/1
  [mrst] -> Delay9/1
  [board_id] -> Delay10/1
  Delay31/1 -> packetiser1/1(sync_in)
  Delay6/1 -> packetiser1/2(data_valid)
  Delay30/1 -> packetiser1/3(data_in)
  Delay9/1 -> packetiser1/4(mrst_in)
  Delay10/1 -> packetiser1/5(board_id)
  packetiser1/1(data_out) -> Delay23/1
  packetiser1/2(valid_out) -> Delay11/1
  packetiser1/3(eof) -> Delay18/1
  packetiser1/4(hdr_valid) -> Delay14/1
  packetiser1/7(header) -> Delay29/1
  packetiser1/5(dest_roach_board) -> Delay28/1
  packetiser1/6(discard) -> Delay17/1
  Delay23/1 -> [pkt1_data], data_out1/1
  Delay11/1 -> [pkt1_vld], data_valid1/1
  Delay28/1 -> dest_roach1/1
  Delay18/1 -> eof1/1
  Delay17/1 -> x_packet_err1/1
  Delay14/1 -> [hdr1_vld]
  Delay29/1 -> [hdr1_data]
  ct/9(cal_fail1) -> cal_fail1/1
  new_acc/1(new_acc) -> Gateway Out/1, [new_acc], ct/1(new_acc)
  new_acc/2(use_data) -> Gateway Out1/1, [data_valid], ct/2(valid_in)
  new_acc/3(slot_0) -> Gateway Out2/1, ct/3(slot_0)
  new_acc/4(data_out) -> ct/4(data_in), Slice/1, Slice5/1
  Gateway Out1/1 -> Scope/2
  Gateway Out4/1 -> Scope/5
  Gateway Out2/1 -> Scope/3
  Gateway Out/1 -> Scope/1
  Gateway Out3/1 -> Scope/4
  Slice/1 -> Gateway Out3/1
  Slice5/1 -> Gateway Out4/1
  Gateway Out6/1 -> Scope1/2
  ? -> Scope1/5
  Gateway Out7/1 -> Scope1/3
  Gateway Out5/1 -> Scope1/1
  Gateway Out8/1 -> Scope1/4
  Slice7/1 -> Gateway Out7/1
  Slice6/1 -> Gateway Out8/1
  Gateway Out10/1 -> Scope2/2
  Gateway Out11/1 -> Scope2/3
  Gateway Out9/1 -> Scope2/1
  Gateway Out14/1 -> Scope2/4
  Gateway Out12/1 -> Scope2/5
  Gateway Out13/1 -> Scope2/6
  Gateway Out16/1 -> Scope3/2
  Gateway Out19/1 -> Scope3/5
  Gateway Out17/1 -> Scope3/3
  Gateway Out15/1 -> Scope3/1
  Gateway Out18/1 -> Scope3/4
  Slice8/1 -> Gateway Out15/1
  [trig_reorder] -> Gateway Out14/1
  [ant0_xport0] -> Gateway Out12/1
  [ant0_xport1] -> Gateway Out13/1
  [p0] -> Gateway Out10/1
  [trig_tvg] -> Gateway Out9/1
